simulink model "mahony"  (R2016a)
settings: Solver=VariableStepAuto  StartTime=0.0  StopTime=10.0  RelTol=1e-3
settings Model: Creator=mgreiff  LastModifiedBy=mgreiff

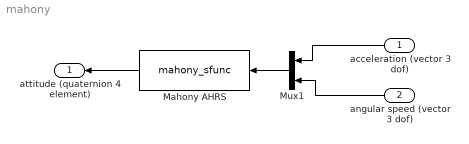
== system mahony ==
  acceleration (vector 3 dof) : Inport  PortDimensions=3
  angular speed (vector 3 dof) : Inport  Port=2  PortDimensions=3
  Mahony AHRS : S-Function  FunctionName=mahony_sfunc  Parameters=MAHparam  SFunctionDeploymentMode=off  EnableBusSupport=off
  Mux1 : Mux  Inputs=2
  attitude (quaternion 4 element) : Outport
  wires:
  acceleration (vector 3 dof)/1 -> Mux1/1
  angular speed (vector 3 dof)/1 -> Mux1/2
  Mahony AHRS/1 -> attitude (quaternion 4 element)/1
  Mux1/1 -> Mahony AHRS/1
